simulink model "bh_SM_quad_and_PEND_obs_explore"  (R2021b)
settings: Solver=ode23t  StartTime=0.0  StopTime=5  FixedStep=0.001  RelTol=1e-5  EnableMultiTasking=on
values from neighbouring files (symbols this model uses):
  K = [-0.0682672734655 -0.00101534451739 0.0236691682063 0.016091917563 -1.50514796185e-07 2.01115560271e-08 -0.0925308250842 6.86252516377e-06 -2.14429477696e-08 -0.092530920783 -3.6011580498e-08 1.11612667422e-06 ... (84 elements, 4x21)]    [CONFIRMED_bh_CONT_DES_RESULTS.mat]
undefined symbols (not defined in the file or in its folder): Continuous, P_elec, P_mot, P_one_prop, P_pend, P_rot, P_veh, P_veh_no_props, sigbuilder_block, Time, X, xme_dot_0, Y, Z
libraries: fl_lib x85, nesl_utility x39, sm_lib x30, simulink_extras x15, fl_ps_legacy_lib x7, slpidlib x4, ctrlSharedLib x1, simulink x1, bh_6dof_LIBRARY x1
(part 4 of 4)

== system bh_SM_quad_and_PEND_obs_explore/MODEL_SYS/bh_6DOF (Simscape)/Propellers/MOT_AERO_PROP_4/DRAQ_and_Thrust_on_PROP ==
  note: The "-1" is because DRAG is in the opposite direction
      | to the propeller SPIN direction
  PS Gain : fl_lib/Physical Signals/Functions/PS Gain  gain=-1
      settings: AttributesFormatString=GAIN= %<gain>
  PS Gain1 : fl_lib/Physical Signals/Functions/PS Gain  gain=P_one_prop.TWIST_per_w2 N*m/((rad/s)^2)
      settings: AttributesFormatString=GAIN= %<gain>
  PS Gain3 : fl_lib/Physical Signals/Functions/PS Gain  gain=P_one_prop.LIFT_per_w2 N/((rad/s)^2)
      settings: AttributesFormatString=GAIN= %<gain>
  PS Product : fl_lib/Physical Signals/Functions/PS Product
  PS Product1 : fl_lib/Physical Signals/Functions/PS Product
  PS Product2 : fl_lib/Physical Signals/Functions/PS Product
  PS Sign : fl_lib/Physical Signals/Nonlinear Operators/PS Sign
      settings: SourceProductBaseCode=SS  InternalSimscapePortConfiguration="{\"Bottom\":[],\"Left\":[{\"id\":\"I\",\"label\":\"\",\"type\":\"input\"}],\"Right\":[{\"id\":\"O\",\"label\":\"\",\"type\":\"output\"}],\"Top\":[]}"
  PS-Simulink Converter1 : nesl_utility/PS-Simulink Converter  PhysicalDomain=network_engine_domain  SubClassName=ps_output  LeftPortType=input  RightPortType=output  PseudoPeriodic=off  Frequencies=[]  Unit=N  AffineConversion=off
      settings: SourceProductBaseCode=PW,SS
  W : PMIOPort  Side=Left
  THRUST : PMIOPort  Port=2  Side=Right
  DRAQ_TQ : PMIOPort  Port=3  Side=Right
  TH_veh : Outport  VectorParamsAs1DForOutWhenUnconnected=off
  wires:
  PS-Simulink Converter1/1 -> TH_veh/1
  connections:
  PS Gain/LConn1 -- PS Sign/RConn1
  W/RConn1 -- PS Product/LConn1 -- PS Product/LConn2 -- PS Product2/LConn1 -- PS Product2/LConn2 -- PS Sign/LConn1
  PS Product/RConn1 -- PS Gain1/LConn1
  PS Gain1/RConn1 -- PS Product1/LConn2
  PS Gain/RConn1 -- PS Product1/LConn1
  DRAQ_TQ/RConn1 -- PS Product1/RConn1
  PS Product2/RConn1 -- PS Gain3/LConn1
  THRUST/RConn1 -- PS Gain3/RConn1 -- PS-Simulink Converter1/LConn1

== system bh_SM_quad_and_PEND_obs_explore/MODEL_SYS/bh_6DOF (Simscape)/Propellers/MOT_AERO_PROP_4/TQ_on_propeller ==
  note: ATTENTION:
      | This subsystem computes the Torque that is applied to the
      | PROPELLER ... and NOT the torque applied to the airframe
  w_CMD_signed : Inport
  DC_mot_elec : Subsystem  mask(DC motor){K=P_mot.Ka, R=P_mot.R, L=P_mot.L, Kb=P_mot.Ke, ID=P_mot.ID}
      mask prompts: K "Torque constant (N.m/A)"; R "Armature resistance (ohms)"; L "Armature Inductance (Henry)"; Kb "Back Emf constant (V.sec/rad)"; ID "Motor_ID  (#1 to #4)"
      mask help: DC motor
      mask DialogControl Container4 Prompt: Mechanical
      mask DialogControl Container9 Prompt: Electrical
      mask DialogControl Container32 Prompt: ID
      mask Display: disp('DC motor')
  DC_mot_elec1 : Subsystem  Commented=on  mask(DC motor){K=P_mot.Ka, R=P_mot.R, L=P_mot.L, Kb=P_mot.Ke, ID=P_mot.ID}
      mask prompts: K "Torque constant (N.m/A)"; R "Armature resistance (ohms)"; L "Armature Inductance (Henry)"; Kb "Back Emf constant (V.sec/rad)"; ID "Motor_ID  (#1 to #4)"
      mask help: DC motor
      mask DialogControl Container4 Prompt: Mechanical
      mask DialogControl Container9 Prompt: Electrical
      mask DialogControl Container32 Prompt: ID
      mask Display: disp('DC motor')
  Mux1 : Mux  Inputs=2
  PI_CONT : slpidlib/PID Controller  Controller=PI  Form=Parallel  TimeDomain=Continuous-time  UseExternalTs=off  SampleTime=-1  IntegratorMethod=Forward Euler  FilterMethod=Forward Euler  ControllerParametersSource=internal  P=2.97678216835849  I=24.9655384194189  D=-0.0417302954853434  UseFilter=on  N=6.67624174583517  TunerSelectOption=Transfer Function Based (PID Tuner App)  InitialConditionSource=internal  InitialConditionForIntegrator=0  InitialConditionForFilter=0  DifferentiatorICPrevScaledInput=0  ExternalReset=none  TrackingMode=off  Kt=1  LimitOutput=off  SatLimitsSource=internal  UpperSaturationLimit=inf  LowerSaturationLimit=-inf  LinearizeAsGain=on  AntiWindupMode=none  Kb=1  POutMin=[]  POutMax=[]  IOutMin=[]  IOutMax=[]  DOutMin=[]  DOutMax=[]  NOutMin=[]  NOutMax=[]  SumOutMin=[]  SumOutMax=[]  SaturationOutMin=[]  SaturationOutMax=[]  PParamMin=[]  PParamMax=[]  IParamMin=[]  IParamMax=[]  DParamMin=[]  DParamMax=[]  NParamMin=[]  NParamMax=[]  KbParamMin=[]  KbParamMax=[]  KtParamMin=[]  KtParamMax=[]  KbOutMin=[]  KbOutMax=[]  KtOutMin=[]  KtOutMax=[]  IntegratorOutMin=[]  IntegratorOutMax=[]  FilterOutMin=[]  FilterOutMax=[]  SumI1OutMin=[]  SumI1OutMax=[]  SumI2OutMin=[]  SumI2OutMax=[]  SumI3OutMin=[]  SumI3OutMax=[]  SumI4OutMin=[]  SumI4OutMax=[]  SumDOutMin=[]  SumDOutMax=[]  DifferentiatorOutMin=[]  DifferentiatorOutMax=[]  FilterDiffOutCoefMin=[]  FilterDiffOutCoefMax=[]  ReciprocalOutMin=[]  ReciprocalOutMax=[]  SumDenOutMin=[]  SumDenOutMax=[]  SumNumOutMin=[]  SumNumOutMax=[]  DivideOutMin=[]  DivideOutMax=[]  UdiffTsProdOutMin=[]  UdiffTsProdOutMax=[]  NTsProdOutMin=[]  NTsProdOutMax=[]  UintegralTsProdOutMin=[]  UintegralTsProdOutMax=[]  UngainTsProdOutMin=[]  UngainTsProdOutMax=[]  IntegratorContinuousStateAttributes=''  IntegratorStateMustResolveToSignalObject=off  IntegratorRTWStateStorageClass=Auto  FilterContinuousStateAttributes=''  FilterStateMustResolveToSignalObject=off  FilterRTWStateStorageClass=Auto  ParallelPVariant=InternalParameters  IdealPVariant=Disabled  IVariant=InternalParameters  DVariant=Disabled  IntegratorVariant=Continuous  SatVariant=Disabled  AWVariant=Passthrough  PCopyVariant=Disabled  TRVariant=Disabled  FdbkBlocksVariant=Forward  IdealPFdbkVariant=Disabled  SatFdbkVariant=Disabled  DerivativeFilterVariant=Disabled  NVariant=Disabled  NCopyVariant=Disabled_SignalSpec  FilterICVariant=Disabled  IntegratorICVariant=InternalICs  ExternalResetVariant=Disabled  TRSumVariant=Passthrough  SumFdbkVariant=Disabled  SumVariant=Sum_PI  TsampFilterVariant=InternalTs  TsampNgainVariant=Passthrough  TsampIntegralVariant=Passthrough  ExternalSaturationOutDataTypeStr=Inherit: Same as second input
  PS-Simulink Converter : nesl_utility/PS-Simulink Converter  PhysicalDomain=network_engine_domain  SubClassName=ps_output  LeftPortType=input  RightPortType=output  PseudoPeriodic=off  Frequencies=[]  Unit=rad/s  AffineConversion=off
      settings: SourceProductBaseCode=PW,SS
  PS-Simulink Converter1 : nesl_utility/PS-Simulink Converter  PhysicalDomain=network_engine_domain  SubClassName=ps_output  LeftPortType=input  RightPortType=output  PseudoPeriodic=off  Frequencies=[]  Unit=N*m  AffineConversion=off
      settings: SourceProductBaseCode=PW,SS
  Scope : Scope
  Simulink-PS Converter2 : nesl_utility/Simulink-PS Converter  PhysicalDomain=network_engine_domain  SubClassName=ps_input  LeftPortType=input  RightPortType=output  PseudoPeriodic=off  Frequencies=[]  NoiseDistribution=none  NoiseParameters=[]  Unit=V  AffineConversion=off  FilteringAndDerivatives=provide  SimscapeFilterOrder=1  InputFilterTimeConstant=0.001  UdotUserProvided=0
      settings: SourceProductBaseCode=PW,SS
  Sum1 : Sum  Inputs=|+-
  VOLTAGE Saturation : Saturate  UpperLimit=P_elec.V_mot_min  LowerLimit=-1*P_elec.V_mot_max
      settings: AttributesFormatString=|
      | Vmax = %<UpperLimit>
      | Vmin = %<LowerLimit>
  VOLTS : Scope
  Ki : PMIOPort  Side=Right
  W_MEAS : PMIOPort  Port=2  Side=Left
  TQ_Ki : Outport  VectorParamsAs1DForOutWhenUnconnected=off
  wires:
  VOLTAGE Saturation/1 -> Simulink-PS Converter2/1, VOLTS/1  "VOLTS"
  Sum1/1 -> PI_CONT/1
  PI_CONT/1 -> VOLTAGE Saturation/1  "VOLTS"
  w_CMD_signed/1 -> Sum1/1, [w_signed]  "w_rad_per_sec"
  PS-Simulink Converter/1 -> [wM], Sum1/2
  PS-Simulink Converter1/1 -> TQ_Ki/1
  Mux1/1 -> Scope/1
  [w_signed] -> Mux1/1
  [wM] -> Mux1/2
  connections:
  DC_mot_elec/LConn1 -- Simulink-PS Converter2/RConn1
  PS-Simulink Converter1/LConn1 -- Ki/RConn1 -- DC_mot_elec/RConn1
  W_MEAS/RConn1 -- PS-Simulink Converter/LConn1 -- DC_mot_elec/LConn2

== system bh_SM_quad_and_PEND_obs_explore/MODEL_SYS/bh_6DOF (Simscape)/Propellers/MOT_AERO_PROP_1/TQ_on_propeller/DC_mot_elec ==
  note: DC Motor - First Principle Equations
  note: L di/dt = V - R i - K_{emf}\fontsize{20}\omega
  PS Constant : fl_lib/Physical Signals/Sources/PS Constant  constant=L H
      settings: AttributesFormatString=|
      | %<constant>
      | UNITS = %<constant_unit>
  PS Divide : fl_lib/Physical Signals/Functions/PS Divide
      settings: SourceProductBaseCode=SS
  PS Gain1 : fl_lib/Physical Signals/Functions/PS Gain  gain=Kb V*s/rad
      settings: AttributesFormatString=|
      | GAIN= %<gain>
      | UNITS = %<gain_unit>
  PS Gain2 : fl_lib/Physical Signals/Functions/PS Gain  gain=R Ohm
      settings: AttributesFormatString=|
      | GAIN= %<gain>
      | UNITS = %<gain_unit>
  PS Gain3 : fl_lib/Physical Signals/Functions/PS Gain  gain=K N*m/A
      settings: AttributesFormatString=|
      | GAIN= %<gain>
      | UNITS = %<gain_unit>
  PS Integrator : fl_lib/Physical Signals/Linear Operators/PS Integrator  reset_method=foundation.enum.IntegratorResetSpec.None  initial_condition_spec=foundation.enum.IntegratorICSpec.Internal  x0=0 A
      settings: AttributesFormatString=UNITS = %<x0_unit>  SourceProductBaseCode=SS
  PS Subtract1 : fl_lib/Physical Signals/Functions/PS Subtract
  PS Subtract2 : fl_lib/Physical Signals/Functions/PS Subtract
  V : PMIOPort  Side=Left
  W : PMIOPort  Port=2  Side=Left
  Ki : PMIOPort  Port=3  Side=Right
  connections:
  PS Subtract1/LConn1 -- V/RConn1
  PS Gain1/RConn1 -- PS Subtract1/LConn2
  W/RConn1 -- PS Gain1/LConn1
  PS Subtract2/LConn1 -- PS Subtract1/RConn1
  PS Gain2/RConn1 -- PS Subtract2/LConn2
  PS Integrator/RConn1 -- PS Gain3/LConn1 -- PS Gain2/LConn1
  PS Divide/RConn1 -- PS Integrator/LConn1
  PS Subtract2/RConn1 -- PS Divide/LConn1
  PS Constant/RConn1 -- PS Divide/LConn2
  Ki/RConn1 -- PS Gain3/RConn1

== system bh_SM_quad_and_PEND_obs_explore/MODEL_SYS/bh_6DOF (Simscape)/Propellers/MOT_AERO_PROP_1/TQ_on_propeller/DC_mot_elec1 ==
  note: DC Motor - First Principle Equations
  note: L di/dt = V - R i - K_{emf}\fontsize{20}\omega
  PS Constant : fl_lib/Physical Signals/Sources/PS Constant  constant=L
      settings: AttributesFormatString=%<constant>
  PS Divide : fl_ps_legacy_lib/Legacy Physical Signals/Functions/PS Divide
      settings: SourceProductBaseCode=SS  InternalSimscapePortConfiguration="{\"Bottom\":[],\"Left\":[{\"id\":\"I1\",\"label\":\"\",\"type\":\"input\"},{\"id\":\"I2\",\"label\":\"\",\"type\":\"input\"}],\"Right\":[{\"id\":\"O\",\"label\":\"\",\"type\":\"output\"}],\"Top\":[]}"
  PS Gain1 : fl_ps_legacy_lib/Legacy Physical Signals/Functions/PS Gain  gain=Kb
      settings: AttributesFormatString=GAIN= %<gain>
  PS Gain2 : fl_ps_legacy_lib/Legacy Physical Signals/Functions/PS Gain  gain=R
      settings: AttributesFormatString=GAIN= %<gain>
  PS Gain3 : fl_ps_legacy_lib/Legacy Physical Signals/Functions/PS Gain  gain=K
      settings: AttributesFormatString=GAIN= %<gain>
  PS Integrator : fl_ps_legacy_lib/Legacy Physical Signals/Linear Operators/PS Integrator  x0=0
      settings: SourceProductBaseCode=SS  InternalSimscapePortConfiguration="{\"Bottom\":[],\"Left\":[{\"id\":\"I\",\"label\":\"\",\"type\":\"input\"}],\"Right\":[{\"id\":\"O\",\"label\":\"\",\"type\":\"output\"}],\"Top\":[]}"
  PS Subtract1 : fl_ps_legacy_lib/Legacy Physical Signals/Functions/PS Subtract
      settings: SourceProductBaseCode=SS
  PS Subtract2 : fl_ps_legacy_lib/Legacy Physical Signals/Functions/PS Subtract
      settings: SourceProductBaseCode=SS
  V : PMIOPort  Side=Left
  W : PMIOPort  Port=2  Side=Left
  Ki : PMIOPort  Port=3  Side=Right
  connections:
  PS Subtract1/LConn1 -- V/RConn1
  PS Gain1/RConn1 -- PS Subtract1/LConn2
  W/RConn1 -- PS Gain1/LConn1
  PS Subtract2/LConn1 -- PS Subtract1/RConn1
  PS Gain2/RConn1 -- PS Subtract2/LConn2
  PS Integrator/RConn1 -- PS Gain3/LConn1 -- PS Gain2/LConn1
  PS Divide/RConn1 -- PS Integrator/LConn1
  PS Subtract2/RConn1 -- PS Divide/LConn1
  PS Constant/RConn1 -- PS Divide/LConn2
  Ki/RConn1 -- PS Gain3/RConn1

== system bh_SM_quad_and_PEND_obs_explore/MODEL_SYS/bh_6DOF (Simscape)/Propellers/MOT_AERO_PROP_2/TQ_on_propeller/DC_mot_elec ==
  note: DC Motor - First Principle Equations
  note: L di/dt = V - R i - K_{emf}\fontsize{20}\omega
  PS Constant : fl_lib/Physical Signals/Sources/PS Constant  constant=L H
      settings: AttributesFormatString=|
      | %<constant>
      | UNITS = %<constant_unit>
  PS Divide : fl_lib/Physical Signals/Functions/PS Divide
      settings: SourceProductBaseCode=SS
  PS Gain1 : fl_lib/Physical Signals/Functions/PS Gain  gain=Kb V*s/rad
      settings: AttributesFormatString=|
      | GAIN= %<gain>
      | UNITS = %<gain_unit>
  PS Gain2 : fl_lib/Physical Signals/Functions/PS Gain  gain=R Ohm
      settings: AttributesFormatString=|
      | GAIN= %<gain>
      | UNITS = %<gain_unit>
  PS Gain3 : fl_lib/Physical Signals/Functions/PS Gain  gain=K N*m/A
      settings: AttributesFormatString=|
      | GAIN= %<gain>
      | UNITS = %<gain_unit>
  PS Integrator : fl_lib/Physical Signals/Linear Operators/PS Integrator  reset_method=foundation.enum.IntegratorResetSpec.None  initial_condition_spec=foundation.enum.IntegratorICSpec.Internal  x0=0 A
      settings: AttributesFormatString=UNITS = %<x0_unit>  SourceProductBaseCode=SS
  PS Subtract1 : fl_lib/Physical Signals/Functions/PS Subtract
  PS Subtract2 : fl_lib/Physical Signals/Functions/PS Subtract
  V : PMIOPort  Side=Left
  W : PMIOPort  Port=2  Side=Left
  Ki : PMIOPort  Port=3  Side=Right
  connections:
  PS Subtract1/LConn1 -- V/RConn1
  PS Gain1/RConn1 -- PS Subtract1/LConn2
  W/RConn1 -- PS Gain1/LConn1
  PS Subtract2/LConn1 -- PS Subtract1/RConn1
  PS Gain2/RConn1 -- PS Subtract2/LConn2
  PS Integrator/RConn1 -- PS Gain3/LConn1 -- PS Gain2/LConn1
  PS Divide/RConn1 -- PS Integrator/LConn1
  PS Subtract2/RConn1 -- PS Divide/LConn1
  PS Constant/RConn1 -- PS Divide/LConn2
  Ki/RConn1 -- PS Gain3/RConn1

== system bh_SM_quad_and_PEND_obs_explore/MODEL_SYS/bh_6DOF (Simscape)/Propellers/MOT_AERO_PROP_2/TQ_on_propeller/DC_mot_elec1 ==
  note: DC Motor - First Principle Equations
  note: L di/dt = V - R i - K_{emf}\fontsize{20}\omega
  PS Constant : fl_lib/Physical Signals/Sources/PS Constant  constant=L
      settings: AttributesFormatString=%<constant>
  PS Divide : fl_lib/Physical Signals/Functions/PS Divide
      settings: SourceProductBaseCode=SS
  PS Gain1 : fl_lib/Physical Signals/Functions/PS Gain  gain=Kb
      settings: AttributesFormatString=GAIN= %<gain>
  PS Gain2 : fl_lib/Physical Signals/Functions/PS Gain  gain=R
      settings: AttributesFormatString=GAIN= %<gain>
  PS Gain3 : fl_lib/Physical Signals/Functions/PS Gain  gain=K
      settings: AttributesFormatString=GAIN= %<gain>
  PS Integrator : fl_lib/Physical Signals/Linear Operators/PS Integrator  x0=0 s
      settings: SourceProductBaseCode=SS
  PS Subtract1 : fl_lib/Physical Signals/Functions/PS Subtract
  PS Subtract2 : fl_lib/Physical Signals/Functions/PS Subtract
  V : PMIOPort  Side=Left
  W : PMIOPort  Port=2  Side=Left
  Ki : PMIOPort  Port=3  Side=Right
  connections:
  PS Subtract1/LConn1 -- V/RConn1
  PS Gain1/RConn1 -- PS Subtract1/LConn2
  W/RConn1 -- PS Gain1/LConn1
  PS Subtract2/LConn1 -- PS Subtract1/RConn1
  PS Gain2/RConn1 -- PS Subtract2/LConn2
  PS Integrator/RConn1 -- PS Gain3/LConn1 -- PS Gain2/LConn1
  PS Divide/RConn1 -- PS Integrator/LConn1
  PS Subtract2/RConn1 -- PS Divide/LConn1
  PS Constant/RConn1 -- PS Divide/LConn2
  Ki/RConn1 -- PS Gain3/RConn1

== system bh_SM_quad_and_PEND_obs_explore/MODEL_SYS/bh_6DOF (Simscape)/Propellers/MOT_AERO_PROP_3/TQ_on_propeller/DC_mot_elec ==
  note: DC Motor - First Principle Equations
  note: L di/dt = V - R i - K_{emf}\fontsize{20}\omega
  PS Constant : fl_lib/Physical Signals/Sources/PS Constant  constant=L H
      settings: AttributesFormatString=|
      | %<constant>
      | UNITS = %<constant_unit>
  PS Divide : fl_lib/Physical Signals/Functions/PS Divide
      settings: SourceProductBaseCode=SS
  PS Gain1 : fl_lib/Physical Signals/Functions/PS Gain  gain=Kb V*s/rad
      settings: AttributesFormatString=|
      | GAIN= %<gain>
      | UNITS = %<gain_unit>
  PS Gain2 : fl_lib/Physical Signals/Functions/PS Gain  gain=R Ohm
      settings: AttributesFormatString=|
      | GAIN= %<gain>
      | UNITS = %<gain_unit>
  PS Gain3 : fl_lib/Physical Signals/Functions/PS Gain  gain=K N*m/A
      settings: AttributesFormatString=|
      | GAIN= %<gain>
      | UNITS = %<gain_unit>
  PS Integrator : fl_lib/Physical Signals/Linear Operators/PS Integrator  reset_method=foundation.enum.IntegratorResetSpec.None  initial_condition_spec=foundation.enum.IntegratorICSpec.Internal  x0=0 A
      settings: AttributesFormatString=UNITS = %<x0_unit>  SourceProductBaseCode=SS
  PS Subtract1 : fl_lib/Physical Signals/Functions/PS Subtract
  PS Subtract2 : fl_lib/Physical Signals/Functions/PS Subtract
  V : PMIOPort  Side=Left
  W : PMIOPort  Port=2  Side=Left
  Ki : PMIOPort  Port=3  Side=Right
  connections:
  PS Subtract1/LConn1 -- V/RConn1
  PS Gain1/RConn1 -- PS Subtract1/LConn2
  W/RConn1 -- PS Gain1/LConn1
  PS Subtract2/LConn1 -- PS Subtract1/RConn1
  PS Gain2/RConn1 -- PS Subtract2/LConn2
  PS Integrator/RConn1 -- PS Gain3/LConn1 -- PS Gain2/LConn1
  PS Divide/RConn1 -- PS Integrator/LConn1
  PS Subtract2/RConn1 -- PS Divide/LConn1
  PS Constant/RConn1 -- PS Divide/LConn2
  Ki/RConn1 -- PS Gain3/RConn1

== system bh_SM_quad_and_PEND_obs_explore/MODEL_SYS/bh_6DOF (Simscape)/Propellers/MOT_AERO_PROP_3/TQ_on_propeller/DC_mot_elec1 ==
  note: DC Motor - First Principle Equations
  note: L di/dt = V - R i - K_{emf}\fontsize{20}\omega
  PS Constant : fl_lib/Physical Signals/Sources/PS Constant  constant=L
      settings: AttributesFormatString=%<constant>
  PS Divide : fl_lib/Physical Signals/Functions/PS Divide
      settings: SourceProductBaseCode=SS
  PS Gain1 : fl_lib/Physical Signals/Functions/PS Gain  gain=Kb
      settings: AttributesFormatString=GAIN= %<gain>
  PS Gain2 : fl_lib/Physical Signals/Functions/PS Gain  gain=R
      settings: AttributesFormatString=GAIN= %<gain>
  PS Gain3 : fl_lib/Physical Signals/Functions/PS Gain  gain=K
      settings: AttributesFormatString=GAIN= %<gain>
  PS Integrator : fl_lib/Physical Signals/Linear Operators/PS Integrator  reset_method=foundation.enum.IntegratorResetSpec.None  initial_condition_spec=foundation.enum.IntegratorICSpec.Internal  x0=0 s
      settings: SourceProductBaseCode=SS
  PS Subtract1 : fl_lib/Physical Signals/Functions/PS Subtract
  PS Subtract2 : fl_lib/Physical Signals/Functions/PS Subtract
  V : PMIOPort  Side=Left
  W : PMIOPort  Port=2  Side=Left
  Ki : PMIOPort  Port=3  Side=Right
  connections:
  PS Subtract1/LConn1 -- V/RConn1
  PS Gain1/RConn1 -- PS Subtract1/LConn2
  W/RConn1 -- PS Gain1/LConn1
  PS Subtract2/LConn1 -- PS Subtract1/RConn1
  PS Gain2/RConn1 -- PS Subtract2/LConn2
  PS Integrator/RConn1 -- PS Gain3/LConn1 -- PS Gain2/LConn1
  PS Divide/RConn1 -- PS Integrator/LConn1
  PS Subtract2/RConn1 -- PS Divide/LConn1
  PS Constant/RConn1 -- PS Divide/LConn2
  Ki/RConn1 -- PS Gain3/RConn1

== system bh_SM_quad_and_PEND_obs_explore/MODEL_SYS/bh_6DOF (Simscape)/Propellers/MOT_AERO_PROP_4/TQ_on_propeller/DC_mot_elec ==
  note: DC Motor - First Principle Equations
  note: L di/dt = V - R i - K_{emf}\fontsize{20}\omega
  PS Constant : fl_lib/Physical Signals/Sources/PS Constant  constant=L H
      settings: AttributesFormatString=|
      | %<constant>
      | UNITS = %<constant_unit>
  PS Divide : fl_lib/Physical Signals/Functions/PS Divide
      settings: SourceProductBaseCode=SS
  PS Gain1 : fl_lib/Physical Signals/Functions/PS Gain  gain=Kb V*s/rad
      settings: AttributesFormatString=|
      | GAIN= %<gain>
      | UNITS = %<gain_unit>
  PS Gain2 : fl_lib/Physical Signals/Functions/PS Gain  gain=R Ohm
      settings: AttributesFormatString=|
      | GAIN= %<gain>
      | UNITS = %<gain_unit>
  PS Gain3 : fl_lib/Physical Signals/Functions/PS Gain  gain=K N*m/A
      settings: AttributesFormatString=|
      | GAIN= %<gain>
      | UNITS = %<gain_unit>
  PS Integrator : fl_lib/Physical Signals/Linear Operators/PS Integrator  reset_method=foundation.enum.IntegratorResetSpec.None  initial_condition_spec=foundation.enum.IntegratorICSpec.Internal  x0=0 A
      settings: AttributesFormatString=UNITS = %<x0_unit>  SourceProductBaseCode=SS
  PS Subtract1 : fl_lib/Physical Signals/Functions/PS Subtract
  PS Subtract2 : fl_lib/Physical Signals/Functions/PS Subtract
  V : PMIOPort  Side=Left
  W : PMIOPort  Port=2  Side=Left
  Ki : PMIOPort  Port=3  Side=Right
  connections:
  PS Subtract1/LConn1 -- V/RConn1
  PS Gain1/RConn1 -- PS Subtract1/LConn2
  W/RConn1 -- PS Gain1/LConn1
  PS Subtract2/LConn1 -- PS Subtract1/RConn1
  PS Gain2/RConn1 -- PS Subtract2/LConn2
  PS Integrator/RConn1 -- PS Gain3/LConn1 -- PS Gain2/LConn1
  PS Divide/RConn1 -- PS Integrator/LConn1
  PS Subtract2/RConn1 -- PS Divide/LConn1
  PS Constant/RConn1 -- PS Divide/LConn2
  Ki/RConn1 -- PS Gain3/RConn1

== system bh_SM_quad_and_PEND_obs_explore/MODEL_SYS/bh_6DOF (Simscape)/Propellers/MOT_AERO_PROP_4/TQ_on_propeller/DC_mot_elec1 ==
  note: DC Motor - First Principle Equations
  note: L di/dt = V - R i - K_{emf}\fontsize{20}\omega
  PS Constant : fl_lib/Physical Signals/Sources/PS Constant  constant=L
      settings: AttributesFormatString=%<constant>
  PS Divide : fl_lib/Physical Signals/Functions/PS Divide
      settings: SourceProductBaseCode=SS
  PS Gain1 : fl_lib/Physical Signals/Functions/PS Gain  gain=Kb
      settings: AttributesFormatString=GAIN= %<gain>
  PS Gain2 : fl_lib/Physical Signals/Functions/PS Gain  gain=R
      settings: AttributesFormatString=GAIN= %<gain>
  PS Gain3 : fl_lib/Physical Signals/Functions/PS Gain  gain=K
      settings: AttributesFormatString=GAIN= %<gain>
  PS Integrator : fl_lib/Physical Signals/Linear Operators/PS Integrator  x0=0 s
      settings: SourceProductBaseCode=SS
  PS Subtract1 : fl_lib/Physical Signals/Functions/PS Subtract
  PS Subtract2 : fl_lib/Physical Signals/Functions/PS Subtract
  V : PMIOPort  Side=Left
  W : PMIOPort  Port=2  Side=Left
  Ki : PMIOPort  Port=3  Side=Right
  connections:
  PS Subtract1/LConn1 -- V/RConn1
  PS Gain1/RConn1 -- PS Subtract1/LConn2
  W/RConn1 -- PS Gain1/LConn1
  PS Subtract2/LConn1 -- PS Subtract1/RConn1
  PS Gain2/RConn1 -- PS Subtract2/LConn2
  PS Integrator/RConn1 -- PS Gain3/LConn1 -- PS Gain2/LConn1
  PS Divide/RConn1 -- PS Integrator/LConn1
  PS Subtract2/RConn1 -- PS Divide/LConn1
  PS Constant/RConn1 -- PS Divide/LConn2
  Ki/RConn1 -- PS Gain3/RConn1

== matlab function bh_SM_quad_and_PEND_obs_explore/MODEL_SYS/bh_6DOF (Simscape)/6DOF_JOINT_SYS/Angular_MEAS/calc_DCM ==
  data: bRg input; eul_vec output
function eul_vec = calc_eul_ang(bRg)
%#codegen

% bRg = [ ...
%                               cos(phi)*cos(theta),                              cos(theta)*sin(phi),         -sin(theta);
%  cos(phi)*sin(psi)*sin(theta) - cos(psi)*sin(phi), cos(phi)*cos(psi) + sin(phi)*sin(psi)*sin(theta), cos(theta)*sin(psi);
%  sin(phi)*sin(psi) + cos(phi)*cos(psi)*sin(theta), cos(psi)*sin(phi)*sin(theta) - cos(phi)*sin(psi), cos(psi)*cos(theta);
%  ];

%phi, theta, psi


theta = asin( -bRg(1,3)  ); %  theta is in the range [-pi/2, pi/2]

% Recall the DOC on atan2()
%     atan2(Y,X) is the four quadrant arctangent of the elements of X and Y
%     such that -pi <= atan2(Y,X) <= pi

Y   = bRg(1,2);
X   = bRg(1,1);
phi = atan2(Y,X);

Y   = bRg(2,3);
X   = bRg(3,3);
psi = atan2(Y,X);

% now populate the output
eul_vec    = zeros(3,1);

eul_vec(1) = phi;
eul_vec(2) = theta;
eul_vec(3) = psi;

end

== matlab function bh_SM_quad_and_PEND_obs_explore/MODEL_SYS/bh_6DOF (Simscape)/PEND_SYS/Pend_Angular_MEAS/Calc Euler_rates/my_euler_rates ==
  data: theta input; euler_rates output; psi input; p input; q input; r input
function euler_rates = my_euler_rates(theta,psi,p,q,r)
%#codegen

%    This function was generated by the Symbolic Math Toolbox version 7.0.
%    09-Jun-2016 10:28:25

euler_rates = [(r.*cos(psi)+q.*sin(psi))./cos(theta);
                q.*cos(psi)-r.*sin(psi);
               (p.*cos(theta)+r.*cos(psi).*sin(theta)+q.*sin(psi).*sin(theta))./cos(theta)];

== matlab function bh_SM_quad_and_PEND_obs_explore/MODEL_SYS/bh_6DOF (Simscape)/PEND_SYS/Pend_Angular_MEAS/calc_DCM ==
  data: bRg input; eul_vec output
function eul_vec = calc_eul_ang(bRg)
%#codegen

% bRg = [ ...
%                               cos(phi)*cos(theta),                              cos(theta)*sin(phi),         -sin(theta);
%  cos(phi)*sin(psi)*sin(theta) - cos(psi)*sin(phi), cos(phi)*cos(psi) + sin(phi)*sin(psi)*sin(theta), cos(theta)*sin(psi);
%  sin(phi)*sin(psi) + cos(phi)*cos(psi)*sin(theta), cos(psi)*sin(phi)*sin(theta) - cos(phi)*sin(psi), cos(psi)*cos(theta);
%  ];

%phi, theta, psi


theta = asin( -bRg(1,3)  ); %  theta is in the range [-pi/2, pi/2]

% Recall the DOC on atan2()
%     atan2(Y,X) is the four quadrant arctangent of the elements of X and Y
%     such that -pi <= atan2(Y,X) <= pi

Y   = bRg(1,2);
X   = bRg(1,1);
phi = atan2(Y,X);

Y   = bRg(2,3);
X   = bRg(3,3);
psi = atan2(Y,X);

% now populate the output
eul_vec    = zeros(3,1);

eul_vec(1) = phi;
eul_vec(2) = theta;
eul_vec(3) = psi;

end

== matlab function bh_SM_quad_and_PEND_obs_explore/CONT_SYS W_MOT_CMDS2/w2toFM1 ==
  data: L input; Tbz_col output; Thrust_const input; Twist_const input; w2_col input; Mbz_col output; wM_col output
function [Tbz_col, Mbz_col, wM_col] = w2toFM(L, Thrust_const, Twist_const, w2_col)
%#codegen

    % simplify the variable names
    b = Thrust_const;
    k = Twist_const;

    % construct the co-efficient matrix:
    %  F_and_M = C * w^2
    
%     C = [     b,    b,    b,    b;
%               0,    b*L,  0,   -b*L;
%              -b*L,  0,    b*L,  0;
%              -k,    k,   -k,    k; ];

    Tbz_col = [ b; b; b; b ]  .*  w2_col;     
    Mbz_col = [-k; k;-k; k ]  .*  w2_col;          
    wM_col  = [ 1;-1; 1;-1 ]  .*  sqrt(w2_col); 
end

== matlab function bh_SM_quad_and_PEND_obs_explore/ASSESS_OBSERVER_PERFORMANCE/PLOT_X_Xest/MATLAB Function ==
  data: X_EST input; y1 output; X_true input; y2 output; y3 output; y4 output; y5 output; y6 output; y7 output; y8 output; y9 output; y10 output; y11 output; y12 output; y13 output; y14 output; y15 output; y16 output; y17 output; y18 output
function [y1,y2,y3,y4,y5,y6,y7,y8,y9, y10,y11, y12,y13,y14,y15,y16, y17, y18] = fcn(X_EST, X_true)

    kk=1;   y1 = [X_true(kk); X_EST(kk)];
    kk=2;   y2 = [X_true(kk); X_EST(kk)];
    kk=3;   y3 = [X_true(kk); X_EST(kk)];
    kk=4;   y4 = [X_true(kk); X_EST(kk)];
    kk=5;   y5 = [X_true(kk); X_EST(kk)];
    kk=6;   y6 = [X_true(kk); X_EST(kk)];
    kk=7;   y7 = [X_true(kk); X_EST(kk)];
    kk=8;   y8 = [X_true(kk); X_EST(kk)];   
    kk= 9;  y9 = [X_true(kk); X_EST(kk)];

    kk=10; y10 = [X_true(kk); X_EST(kk)];
    kk=11; y11 = [X_true(kk); X_EST(kk)];
    kk=12; y12 = [X_true(kk); X_EST(kk)];
    kk=13; y13 = [X_true(kk); X_EST(kk)];
    kk=14; y14 = [X_true(kk); X_EST(kk)];
    kk=15; y15 = [X_true(kk); X_EST(kk)];
    kk=16; y16 = [X_true(kk); X_EST(kk)];
    kk=17; y17 = [X_true(kk); X_EST(kk)];
    kk=18; y18 = [X_true(kk); X_EST(kk)];
end

== matlab function bh_SM_quad_and_PEND_obs_explore/CONT_SYS W_MOT_CMDS2/FM_to_w2 ==
  data: L input; w2_cmd output; Thrust_const input; Twist_const input; Thrust input; TQ_roll_X input; TQ_pit_Y input; TQ_yaw_Z input
function w2_cmd = FMtow2(L, Thrust_const, Twist_const, Thrust, TQ_roll_X, TQ_pit_Y, TQ_yaw_Z)
%#codegen

    % simplify the variable names
    b = Thrust_const;
    k = Twist_const;

    % construct the co-efficient matrix:
    %  F_and_M = C * w^2
    %
    C = [     b,    b,    b,    b;
              0,    b*L,  0,   -b*L;
             -b*L,  0,    b*L,  0;
             -k,    k,   -k,    k; ];

    % used Symbolic toolbox to compute inv(C)
    C_inv = [
             1/(4*b),          0, -1/(2*L*b), -1/(4*k);
             1/(4*b),  1/(2*L*b),          0,  1/(4*k);
             1/(4*b),          0,  1/(2*L*b), -1/(4*k);
             1/(4*b), -1/(2*L*b),          0,  1/(4*k);
            ];
    % solve for the w^2 vec
    F_and_M_col = [Thrust, TQ_roll_X, TQ_pit_Y, TQ_yaw_Z].' ;
    w2_cmd      = C_inv * F_and_M_col; 
    % check that ALL w^2 >=0
    tf_col      = (w2_cmd >= 0);
%     if( ~all(tf_col) )
%         w2_cmd = lsqnonneg(C, F_and_M_col);
%     end
%     
%     tf_again_col = (w2_cmd >= 0);
%     assert(all(tf_again_col), 'ERROR: ohh dear some w2 are NEGATIVE !')
   
%     for kk=1:4
%       fprintf('\n ... [%.16f]', w2_cmd(kk) );
%     end
%     fprintf('\n -----------------------------------------------');
    assert(all(tf_col), 'ERROR: ohh dear some w2 are NEGATIVE !')
    
% 
%      if( ~all(tf_col) )
%        fprintf('\n ..... WHAT HAPPENED !');
%      end
%     assert(all(tf_col), 'ERROR: ohh dear some w2 are NEGATIVE !')
   %assert(false, 'ERROR: some w2 are NEGATIVE !')
end

== matlab function bh_SM_quad_and_PEND_obs_explore/a_circle1/MATLAB Function ==
  data: t_clock input; XYZ output; t_to_start input; RADIUS input; ztgt input; w input
function XYZ = fcn(t_clock, t_to_start, RADIUS, ztgt, w)

t    = t_clock - t_to_start;

theta = w*t;

x = RADIUS * cos(theta);
y = RADIUS * sin(theta);
z = ztgt;


XYZ = [x;y;z];

== matlab function bh_SM_quad_and_PEND_obs_explore/ASSESS_OBSERVER_PERFORMANCE/PLOT_Y_Yest/MATLAB Function ==
  data: EST input; y1 output; MEAS input; y2 output; y3 output; y4 output; y5 output; y6 output; y7 output; y8 output; y9 output
function [y1,y2,y3,y4,y5,y6,y7,y8,y9] = fcn(EST, MEAS)

kk=1; y1 = [MEAS(kk); EST(kk)];
kk=2; y2 = [MEAS(kk); EST(kk)];
kk=3; y3 = [MEAS(kk); EST(kk)];

kk=4; y4 = [MEAS(kk); EST(kk)];
kk=5; y5 = [MEAS(kk); EST(kk)];
kk=6; y6 = [MEAS(kk); EST(kk)];

kk=7; y7 = [MEAS(kk); EST(kk)];
kk=8; y8 = [MEAS(kk); EST(kk)];
kk=9; y9 = [MEAS(kk); EST(kk)];

end

== matlab function bh_SM_quad_and_PEND_obs_explore/MODEL_SYS/bh_6DOF (Simscape)/6DOF_JOINT_SYS/Angular_MEAS/Calc Euler_rates/my_euler_rates ==
  data: theta input; euler_rates output; psi input; p input; q input; r input
function euler_rates = my_euler_rates(theta,psi,p,q,r)
%#codegen

%    This function was generated by the Symbolic Math Toolbox version 7.0.
%    09-Jun-2016 10:28:25

euler_rates = [(r.*cos(psi)+q.*sin(psi))./cos(theta);
                q.*cos(psi)-r.*sin(psi);
               (p.*cos(theta)+r.*cos(psi).*sin(theta)+q.*sin(psi).*sin(theta))./cos(theta)];
